simulink model "ex_08_model"  (R2014a)
settings: Solver=ode45  StartTime=0.0  StopTime=10.0  RelTol=1e-3
values from neighbouring files (symbols this model uses):
  G = 0    [ex_08_init.m]    (also in ex_08_plot.m = 0.01)
  Kp = y    (= 400)    [ex_08_init.m]    (also in ex_08_plot.m = 0.5*(-(y/x)))
  x = -(1/J) * (a + (K^2/R))    (= -20.4)    [ex_08_init.m]
  y = (K/(J*R))    (= 400)    [ex_08_init.m]
  z = -(1/J)    (= -4000)    [ex_08_init.m]
settings Model: Creator=Nino  LastModifiedBy=Nino

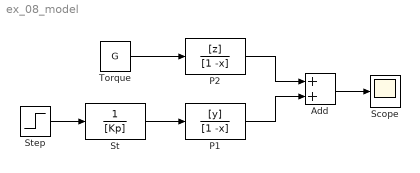
== system ex_08_model ==
  Add : Sum
  P1 : TransferFcn  Numerator=[y]  Denominator=[1 -x]
  P2 : TransferFcn  Numerator=[z]  Denominator=[1 -x]
  Scope : Scope
  St : TransferFcn  Denominator=[Kp]
  Step : Step  After=10  SampleTime=0
  Torque : Constant  Value=G
  wires:
  Add/1 -> Scope/1
  Torque/1 -> P2/1
  P2/1 -> Add/1
  P1/1 -> Add/2
  St/1 -> P1/1
  Step/1 -> St/1
